simulink library "lib_power_bus2"  (Simulink 10.1)
settings: Solver=VariableStepAuto  StartTime=0.0  StopTime=10.0  RelTol=1e-3
undefined symbols (not defined in the file or in its folder): acc_elec_eff, acc_elec_pwr, cs_hi_soc, cs_lo_soc, ess_on
undefined symbols (not defined in the file): logFlag
libraries: sub_lib_models x2
settings Model: Creator=sateeshk  LastModifiedBy=sateeshk
settings Model: ModifiedComment=|
  | mokeefe -- Thu Apr 18 08:38:09 2002 -- Version 1.10
  | saving the model:
  | o "without the model browser open"
  | o with only top-level screen visible
  | o with "fit to view" enabled
  | o with "status bar" off and "toolbar" off
  | o with "prompt to update model history with each save" on
settings Model: ModifiedHistory=|
  | mokeefe -- Thu Apr 18 08:38:09 2002 -- Version 1.10
  | saving the model:
  | o "without the model browser open"
  | o with only top-level screen visible
  | o with "fit to view" enabled
  | o with "status bar" off and "toolbar" off
  | o with "prompt to update model history with each save" on
  | 
  | mokeefe -- Thu Apr 18 08:38:09 2002 -- Version 1.10
  | saving the model:
  | o "without the model browser open"
  | o with only top-level screen visible
  | o with "fit to view" enabled
  | o with "status bar" off and "toolbar" off
  | o with "prompt to update model history with each save" on

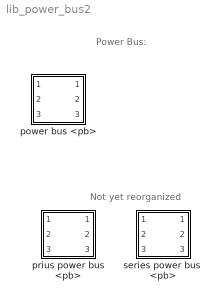
== system lib_power_bus2 ==
  note: Power Bus:
  note: Not yet reorganized
  power bus <pb> : Subsystem  mask(Stand-Alone Power Bus Mask){generalName='pb', logPick=Log, initFileName={}, modCell={}, imgFileName='bdi_pb.jpg', DEBUG=ON}
      mask prompts: generalName "General Name of this Component [char]"; logPick "Log Variables to Workspace?"; initFileName "Initialization File(s) [cell array of char]"; modCell "Modification Cell [2 column cell array of param and val]"; imgFileName "Icon image file name [char--evaluated]"
      mask init:
      | % initialization via m-file script
      | advSACompMaskInit;
      mask TypeOptions logPick: Don't Log | Log
      mask TypeOptions DEBUG: ON | OFF
      mask Display: image(imread(imgFileName))
  prius power bus <pb> : Subsystem
      mask Display: image(imread('bdi_pb.jpg'))
  series power bus  <pb> : Subsystem
      mask Display: image(imread('bdi_pb.jpg'))

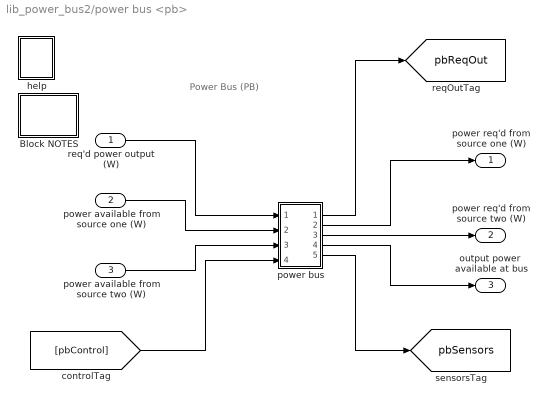
== system lib_power_bus2/power bus <pb> ==
  note: Power Bus (PB)
  req'd power output (W) : Inport
  power available from source one (W) : Inport  Port=2
  power available from source two (W) : Inport  Port=3
  Block NOTES : Subsystem
      mask Display: disp('Block\nNOTES')
  help : Subsystem
      settings: OpenFcn=web(['file:\\\' which('fuel_converter.htm')]);
      mask Display: image(imread('doc_man.jpg'))
  power bus : Subsystem
  power req'd from source one (W) : Outport
  power req'd from source two (W) : Outport  Port=2
  output power  available at bus : Outport  Port=3
  tag scope: pbReqOut=global, pbSensors=global
  wires:
  req'd power output (W)/1 -> power bus/1(power out req)
  power available from source one (W)/1 -> power bus/2(power available from source one)
  power available from source two (W)/1 -> power bus/3(power available from source two)
  [pbControl] -> power bus/4(control)
  power bus/1(required out) -> [pbReqOut]
  power bus/2(power in req from  source one) -> power req'd from source one (W)/1
  power bus/3(power in req from  source two) -> power req'd from source two (W)/1
  power bus/4(power out available) -> output power  available at bus/1
  power bus/5(sensors) -> [pbSensors]

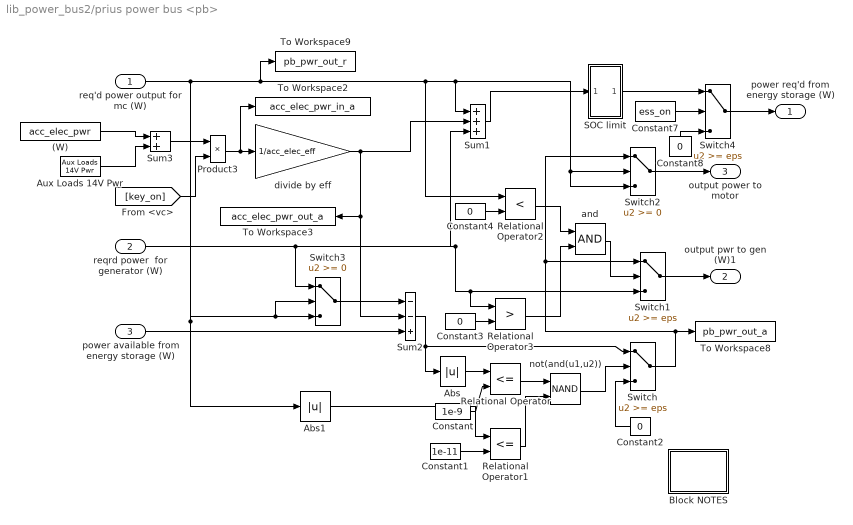
== system lib_power_bus2/prius power bus <pb> ==
  req'd power output for mc (W) : Inport
  reqrd power  for generator (W) : Inport  Port=2
  power available from energy storage (W) : Inport  Port=3
  (W) : Constant  Value=acc_elec_pwr
  Abs : Abs  SaturateOnIntegerOverflow=on
  Abs1 : Abs  SaturateOnIntegerOverflow=on
  Aux Loads 14V Pwr : sub_lib_models/Aux Loads 14V Pwr
      settings: RTWFcnNameOpts=Auto  RTWFileNameOpts=Auto
  Block NOTES : Subsystem
      mask Display: disp('Block\nNOTES')
  Constant : Constant  Value=1e-9
  Constant1 : Constant  Value=1e-11
  Constant{2..4,8} (4 alike) : Constant  Value=0
  Constant7 : Constant  Value=ess_on
  Product3 : Product  SaturateOnIntegerOverflow=on
  Relational Operator : RelationalOperator  Operator=<=  RndMeth=Nearest  InputSameDT=on
  Relational Operator1 : RelationalOperator  Operator=<=  RndMeth=Nearest  InputSameDT=on
  Relational Operator2 : RelationalOperator  Operator=<  RndMeth=Nearest  InputSameDT=on
  Relational Operator3 : RelationalOperator  Operator=>  RndMeth=Nearest  InputSameDT=on
  SOC limit : Subsystem
  Sum1 : Sum  Inputs=+++  SaturateOnIntegerOverflow=on
  Sum2 : Sum  Inputs=--+  SaturateOnIntegerOverflow=on
  Sum3 : Sum  SaturateOnIntegerOverflow=on
  Switch : Switch  Threshold=eps  SaturateOnIntegerOverflow=on  InputSameDT=on
  Switch1 : Switch  Threshold=eps  SaturateOnIntegerOverflow=on  InputSameDT=on
  Switch2 : Switch  SaturateOnIntegerOverflow=on  InputSameDT=on
  Switch3 : Switch  SaturateOnIntegerOverflow=on  InputSameDT=on
  Switch4 : Switch  Threshold=eps  SaturateOnIntegerOverflow=on  InputSameDT=on
  To Workspace2 : ToWorkspace  VariableName=acc_elec_pwr_in_a  SampleTime=-1
  To Workspace3 : ToWorkspace  VariableName=acc_elec_pwr_out_a  SampleTime=-1
  To Workspace8 : ToWorkspace  VariableName=pb_pwr_out_a  SampleTime=-1
  To Workspace9 : ToWorkspace  VariableName=pb_pwr_out_r  SampleTime=-1
  and : Logic
  divide by eff : Gain  Gain=1/acc_elec_eff  SaturateOnIntegerOverflow=on
  not(and(u1,u2)) : Logic  Operator=NAND
  power req'd from energy storage (W) : Outport
  output pwr to gen (W)1 : Outport  Port=2
  output power to motor : Outport  Port=3
  wires:
  and/1 -> Switch1/2
  Relational Operator3/1 -> and/2
  Relational Operator2/1 -> and/1
  Constant4/1 -> Relational Operator2/2
  Constant3/1 -> Relational Operator3/2
  Constant8/1 -> Switch4/3
  Constant7/1 -> Switch4/2
  Switch4/1 -> power req'd from energy storage (W)/1
  SOC limit/1(limited pwr req from ess (W)) -> Switch4/1
  Sum1/1 -> SOC limit/1(pwr req to  ess)
  Switch/1 -> Switch2/1, Switch1/1, To Workspace8/1
  reqrd power  for generator (W)/1 -> Switch3/1, Switch1/3, Relational Operator3/1, Sum1/3
  Switch3/1 -> Sum2/1
  Switch1/1 -> output pwr to gen (W)1/1
  Switch2/1 -> output power to motor/1
  Constant1/1 -> Relational Operator1/2
  Relational Operator1/1 -> not(and(u1,u2))/2
  Abs1/1 -> Relational Operator1/1
  Constant/1 -> Relational Operator/2
  Relational Operator/1 -> not(and(u1,u2))/1
  not(and(u1,u2))/1 -> Switch/2
  Constant2/1 -> Switch/3
  Abs/1 -> Relational Operator/1
  Sum2/1 -> Switch/1, Abs/1
  power available from energy storage (W)/1 -> Sum2/3
  Product3/1 -> To Workspace2/1, divide by eff/1
  divide by eff/1 -> Sum1/2, To Workspace3/1, Sum2/2
  [key_on] -> Product3/2
  req'd power output for mc (W)/1 -> Switch3/2, Switch3/3, Abs1/1, Relational Operator2/1, Switch2/2, Switch2/3, Sum1/1, To Workspace9/1
  Sum3/1 -> Product3/1
  (W)/1 -> Sum3/1
  Aux Loads 14V Pwr/1 -> Sum3/2

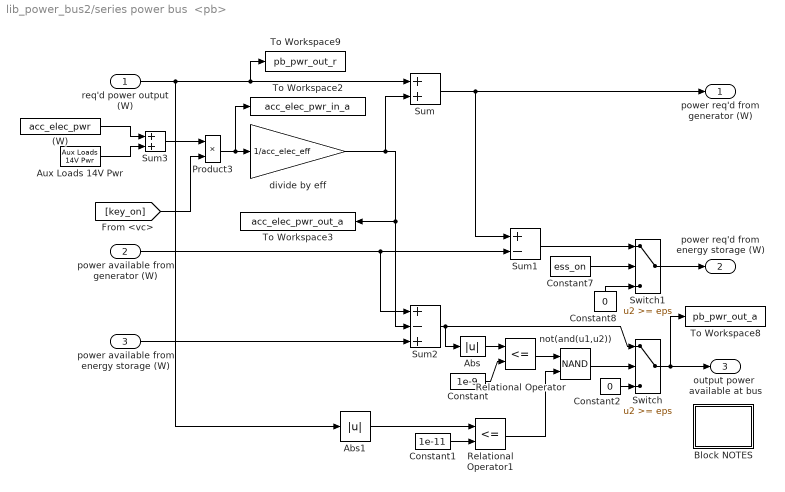
== system lib_power_bus2/series power bus  <pb> ==
  req'd power output (W) : Inport
  power available from generator (W) : Inport  Port=2
  power available from energy storage (W) : Inport  Port=3
  (W) : Constant  Value=acc_elec_pwr
  Abs : Abs  SaturateOnIntegerOverflow=on
  Abs1 : Abs  SaturateOnIntegerOverflow=on
  Aux Loads 14V Pwr : sub_lib_models/Aux Loads 14V Pwr
      settings: RTWFcnNameOpts=Auto  RTWFileNameOpts=Auto
  Block NOTES : Subsystem
      mask Display: disp('Block\nNOTES')
  Constant : Constant  Value=1e-9
  Constant1 : Constant  Value=1e-11
  Constant2 : Constant  Value=0
  Constant7 : Constant  Value=ess_on
  Constant8 : Constant  Value=0
  Product3 : Product  SaturateOnIntegerOverflow=on
  Relational Operator : RelationalOperator  Operator=<=  RndMeth=Nearest  InputSameDT=on
  Relational Operator1 : RelationalOperator  Operator=<=  RndMeth=Nearest  InputSameDT=on
  Sum : Sum  SaturateOnIntegerOverflow=on
  Sum1 : Sum  Inputs=+-  SaturateOnIntegerOverflow=on
  Sum2 : Sum  Inputs=+-+  SaturateOnIntegerOverflow=on
  Sum3 : Sum  SaturateOnIntegerOverflow=on
  Switch : Switch  Threshold=eps  SaturateOnIntegerOverflow=on  InputSameDT=on
  Switch1 : Switch  Threshold=eps  SaturateOnIntegerOverflow=on  InputSameDT=on
  To Workspace2 : ToWorkspace  VariableName=acc_elec_pwr_in_a  SampleTime=-1
  To Workspace3 : ToWorkspace  VariableName=acc_elec_pwr_out_a  SampleTime=-1
  To Workspace8 : ToWorkspace  VariableName=pb_pwr_out_a  SampleTime=-1
  To Workspace9 : ToWorkspace  VariableName=pb_pwr_out_r  SampleTime=-1
  divide by eff : Gain  Gain=1/acc_elec_eff  SaturateOnIntegerOverflow=on
  not(and(u1,u2)) : Logic  Operator=NAND
  power req'd from generator (W) : Outport
  power req'd from energy storage (W) : Outport  Port=2
  output power  available at bus : Outport  Port=3
  wires:
  Constant8/1 -> Switch1/3
  Constant7/1 -> Switch1/2
  Switch1/1 -> power req'd from energy storage (W)/1
  Sum1/1 -> Switch1/1
  Constant/1 -> Relational Operator/2
  Abs/1 -> Relational Operator/1
  Sum2/1 -> Switch/1, Abs/1
  Switch/1 -> output power  available at bus/1, To Workspace8/1
  Constant1/1 -> Relational Operator1/2
  Abs1/1 -> Relational Operator1/1
  Relational Operator1/1 -> not(and(u1,u2))/2
  not(and(u1,u2))/1 -> Switch/2
  Constant2/1 -> Switch/3
  power available from energy storage (W)/1 -> Sum2/3
  Relational Operator/1 -> not(and(u1,u2))/1
  power available from generator (W)/1 -> Sum1/2, Sum2/1
  Product3/1 -> To Workspace2/1, divide by eff/1
  [key_on] -> Product3/2
  Sum/1 -> power req'd from generator (W)/1, Sum1/1
  req'd power output (W)/1 -> To Workspace9/1, Sum/1, Abs1/1
  divide by eff/1 -> Sum/2, Sum2/2, To Workspace3/1
  Sum3/1 -> Product3/1
  (W)/1 -> Sum3/1
  Aux Loads 14V Pwr/1 -> Sum3/2

== system lib_power_bus2/power bus <pb>/Block NOTES ==
  note: This block models the internal combustion engine, and includes inertia effects,
      | performance limits, accessory loads, and temperature transient effects on fuel
      | use, engine-out emissions, and catalyst efficiency.  There are 'leads' to the
      | engine controller here, which controller determines whether the engine is on.

== system lib_power_bus2/power bus <pb>/help ==

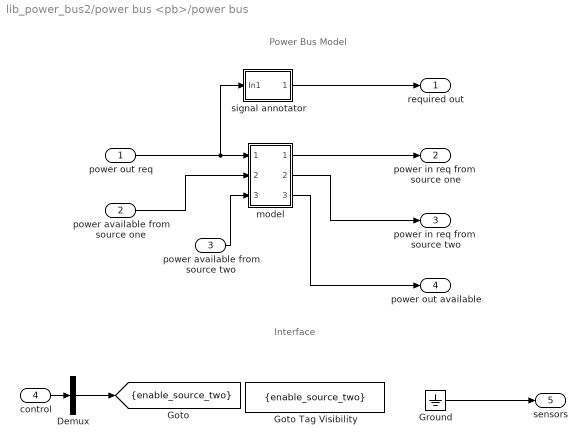
== system lib_power_bus2/power bus <pb>/power bus ==
  note: Interface
  note: Power Bus Model
  power out req : Inport
  power available from source one : Inport  Port=2
  power available from source two : Inport  Port=3
  control : Inport  Port=4
  Demux : Demux  Outputs=1
  Goto Tag Visibility : GotoTagVisibility  GotoTag=enable_source_two
  Ground : Ground
  model : Subsystem
  signal annotator : Subsystem
  required out : Outport
  power in req from  source one : Outport  Port=2
  power in req from  source two : Outport  Port=3
  power out available : Outport  Port=4
  sensors : Outport  Port=5
  tag scope: enable_source_two=scoped
  wires:
  model/1(power req'd from generator (W)) -> power in req from  source one/1
  power out req/1 -> model/1(req'd power output (W)), signal annotator/1(In1)
  model/2(power req'd from energy storage (W)) -> power in req from  source two/1
  power available from source one/1 -> model/2(power available from generator (W))
  model/3(output power  available at bus) -> power out available/1
  power available from source two/1 -> model/3(power available from energy storage (W))
  signal annotator/1(Out1) -> required out/1
  control/1 -> Demux/1
  Demux/1 -> [enable_source_two]
  Ground/1 -> sensors/1

== system lib_power_bus2/prius power bus <pb>/Block NOTES ==
  note: This power bus requires power from (or distributes power to)
      | the generator first, taking the balance from the energy
      | storage system.

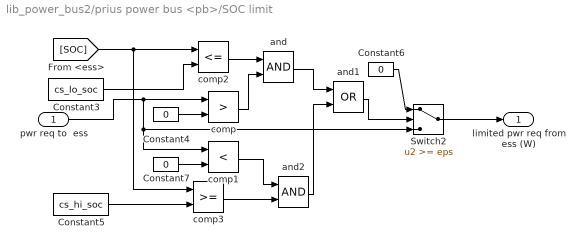
== system lib_power_bus2/prius power bus <pb>/SOC limit ==
  pwr req to  ess : Inport
  Constant3 : Constant  Value=cs_lo_soc
  Constant4 : Constant  Value=0
  Constant5 : Constant  Value=cs_hi_soc
  Constant6 : Constant  Value=0
  Constant7 : Constant  Value=0
  Switch2 : Switch  Threshold=eps  SaturateOnIntegerOverflow=on  InputSameDT=on
  and : Logic
  and1 : Logic  Operator=OR
  and2 : Logic
  comp : RelationalOperator  Operator=>  RndMeth=Nearest  InputSameDT=on
  comp1 : RelationalOperator  Operator=<  RndMeth=Nearest  InputSameDT=on
  comp2 : RelationalOperator  Operator=<=  RndMeth=Nearest  InputSameDT=on
  comp3 : RelationalOperator  RndMeth=Nearest  InputSameDT=on
  limited pwr req from ess (W) : Outport  InitialOutput=0
  wires:
  Switch2/1 -> limited pwr req from ess (W)/1
  comp2/1 -> and/1
  Constant3/1 -> comp2/2
  and/1 -> and1/1
  and1/1 -> Switch2/2
  [SOC] -> comp2/1, comp3/1
  comp/1 -> and/2
  comp1/1 -> and2/1
  pwr req to  ess/1 -> comp/1, comp1/1, Switch2/3
  Constant6/1 -> Switch2/1
  Constant5/1 -> comp3/2
  comp3/1 -> and2/2
  and2/1 -> and1/2
  Constant4/1 -> comp/2
  Constant7/1 -> comp1/2

== system lib_power_bus2/series power bus  <pb>/Block NOTES ==
  note: This power bus requires power from (or distributes power to)
      | the generator first, taking the balance from the energy
      | storage system.

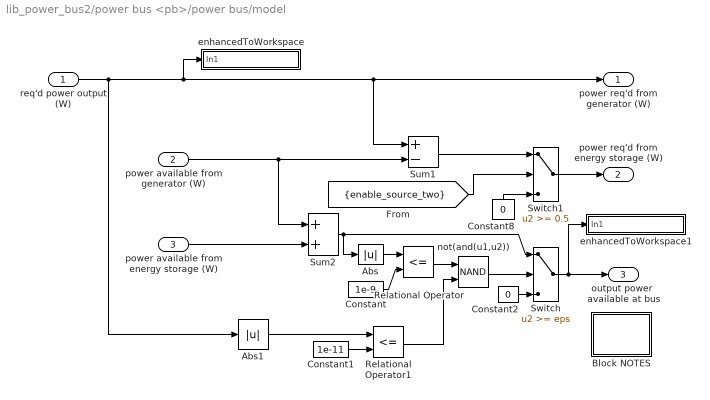
== system lib_power_bus2/power bus <pb>/power bus/model ==
  req'd power output (W) : Inport
  power available from generator (W) : Inport  Port=2
  power available from energy storage (W) : Inport  Port=3
  Abs : Abs  SaturateOnIntegerOverflow=on
  Abs1 : Abs  SaturateOnIntegerOverflow=on
  Block NOTES : Subsystem
      mask Display: disp('Block\nNOTES')
  Constant : Constant  Value=1e-9
  Constant1 : Constant  Value=1e-11
  Constant2 : Constant  Value=0
  Constant8 : Constant  Value=0
  Relational Operator : RelationalOperator  Operator=<=  RndMeth=Nearest  InputSameDT=on
  Relational Operator1 : RelationalOperator  Operator=<=  RndMeth=Nearest  InputSameDT=on
  Sum1 : Sum  Inputs=+-  SaturateOnIntegerOverflow=on
  Sum2 : Sum  SaturateOnIntegerOverflow=on
  Switch : Switch  Threshold=eps  SaturateOnIntegerOverflow=on  InputSameDT=on
  Switch1 : Switch  Threshold=0.5  SaturateOnIntegerOverflow=on  InputSameDT=on
  enhancedToWorkspace : Subsystem  TreatAsAtomicUnit=on  mask(enhancedToWorkspace){generalName=generalName, specificName=pwr_out_r, logFlag=logFlag}
      mask prompts: generalName "General Name [char-evaluated]"; specificName "Specific Name [char-literal]"; logFlag "Enable flag (1=on,0=off)"
      mask help: A wrapper for the Simulink "To Workspace" block that allows you to evaluate the name of the variable to log to workspace. This is useful to avoid the double logging errors that occur when you pull in two library models that attempt to log to the same variable.
      mask init:
      | enhancedToWsMaker
      settings: CopyFcn=breakLinkCopyFcn  ParentCloseFcn=breakLinkParCloseFcn
      mask Help:
      | <h2>Enhanced To Workspace Block</h2>
      | <h3>Parameters</h3>
      | <UL>
      | <li><b>General Name:</b> This is the more general name of the variable. Variables are saved to the workspace as <i>generalName_specificName</i>. Note that this is an evaluated variable. If you would like to type in the value directly, it must be surrounded with single quotes. Otherwise you can input the name of a variable containing a char string.</li>
      | <li><b>Specific Name:</b> This is the specific name of the variable. Note that this is input as a char literal (i.e., you don't need quotes).</li>
      | <li><b>Enable Flag:</b> This flag should have the value of 0 or 1. If 0, the variable will not be logged to the workspace. If 1, the variable will be logged. This is done so that variable logging can be turned off to improve speed.</li>
      | </ul>
      | <h3>Overview</h3>
      | <p>The enhanced to workspace block was put together to allow one to dynamically resolve variable names at run time in simulink. This is most powerful when used in conjunction with a masked subsystem to allow multiple instances of that masked subsytem to be used in the same model. The strategy is to set the generalName in the block mask which will allow the block to change the general name for all variable logging on the fly.
      | <h3>Helper Files</h3>
      | <p>Three m-files are required by the enhancedToWorkspace block. These files are located in the &lt; ADVISOR root &gt;/GUI directory :
      | <ul>
      | <li><i>enhancedToWsMaker.m</i> This file runs the mask initialization for the block</li>
      | <li><i>breakLinkCopyFcn.m</i> This file is used by the block callback when the simulink block is copied. It is necessary to break the link to the enhancedToWorkspace similar to the To Workspace block in order for it to be able to configure itself. (Try copying simulink's To Workspace block--it is impossible to make a link)</li>
      | <li><i>breakLinkParCloseFcn.m</i> This file is similar to the breakLinkCopyFcn and is used when a parent system is closed</li>
      | </ul>
      | <hr>
      | 
      | <p>Created 2003-Jan-21, Michael Patrick O'Keefe, NREL</p>
      | 
      | <!--
      | <VARDEF>
      | <H3>var_name</H3>
      | <UL>
      | <LI><B>data type</B> data type here</LI>
      | <LI><B>units</B> units here</LI>
      | <LI><B>vehicle type</B> vehicle type here</LI>
      | <LI><B>description</B> description here</LI>
      | </UL>
      | </VARDEF>
      | -->
      mask Display: disp([generalName,'_',specificName])
  enhancedToWorkspace1 : Subsystem  TreatAsAtomicUnit=on  mask(enhancedToWorkspace){generalName=generalName, specificName=pwr_out_a, logFlag=logFlag}
      mask prompts: generalName "General Name [char-evaluated]"; specificName "Specific Name [char-literal]"; logFlag "Enable flag (1=on,0=off)"
      mask help: A wrapper for the Simulink "To Workspace" block that allows you to evaluate the name of the variable to log to workspace. This is useful to avoid the double logging errors that occur when you pull in two library models that attempt to log to the same variable.
      mask init:
      | enhancedToWsMaker
      settings: CopyFcn=breakLinkCopyFcn  ParentCloseFcn=breakLinkParCloseFcn
      mask Help:
      | <h2>Enhanced To Workspace Block</h2>
      | <h3>Parameters</h3>
      | <UL>
      | <li><b>General Name:</b> This is the more general name of the variable. Variables are saved to the workspace as <i>generalName_specificName</i>. Note that this is an evaluated variable. If you would like to type in the value directly, it must be surrounded with single quotes. Otherwise you can input the name of a variable containing a char string.</li>
      | <li><b>Specific Name:</b> This is the specific name of the variable. Note that this is input as a char literal (i.e., you don't need quotes).</li>
      | <li><b>Enable Flag:</b> This flag should have the value of 0 or 1. If 0, the variable will not be logged to the workspace. If 1, the variable will be logged. This is done so that variable logging can be turned off to improve speed.</li>
      | </ul>
      | <h3>Overview</h3>
      | <p>The enhanced to workspace block was put together to allow one to dynamically resolve variable names at run time in simulink. This is most powerful when used in conjunction with a masked subsystem to allow multiple instances of that masked subsytem to be used in the same model. The strategy is to set the generalName in the block mask which will allow the block to change the general name for all variable logging on the fly.
      | <h3>Helper Files</h3>
      | <p>Three m-files are required by the enhancedToWorkspace block. These files are located in the &lt; ADVISOR root &gt;/GUI directory :
      | <ul>
      | <li><i>enhancedToWsMaker.m</i> This file runs the mask initialization for the block</li>
      | <li><i>breakLinkCopyFcn.m</i> This file is used by the block callback when the simulink block is copied. It is necessary to break the link to the enhancedToWorkspace similar to the To Workspace block in order for it to be able to configure itself. (Try copying simulink's To Workspace block--it is impossible to make a link)</li>
      | <li><i>breakLinkParCloseFcn.m</i> This file is similar to the breakLinkCopyFcn and is used when a parent system is closed</li>
      | </ul>
      | <hr>
      | 
      | <p>Created 2003-Jan-21, Michael Patrick O'Keefe, NREL</p>
      | 
      | <!--
      | <VARDEF>
      | <H3>var_name</H3>
      | <UL>
      | <LI><B>data type</B> data type here</LI>
      | <LI><B>units</B> units here</LI>
      | <LI><B>vehicle type</B> vehicle type here</LI>
      | <LI><B>description</B> description here</LI>
      | </UL>
      | </VARDEF>
      | -->
      mask Display: disp([generalName,'_',specificName])
  not(and(u1,u2)) : Logic  Operator=NAND
  power req'd from generator (W) : Outport
  power req'd from energy storage (W) : Outport  Port=2
  output power  available at bus : Outport  Port=3
  wires:
  req'd power output (W)/1 -> power req'd from generator (W)/1, Sum1/1, enhancedToWorkspace/1(In1), Abs1/1
  power available from generator (W)/1 -> Sum1/2, Sum2/1
  Relational Operator/1 -> not(and(u1,u2))/1
  Constant2/1 -> Switch/3
  not(and(u1,u2))/1 -> Switch/2
  Relational Operator1/1 -> not(and(u1,u2))/2
  Abs1/1 -> Relational Operator1/1
  Constant1/1 -> Relational Operator1/2
  Switch/1 -> output power  available at bus/1, enhancedToWorkspace1/1(In1)
  Sum2/1 -> Abs/1, Switch/1
  Abs/1 -> Relational Operator/1
  Constant/1 -> Relational Operator/2
  Sum1/1 -> Switch1/1
  Switch1/1 -> power req'd from energy storage (W)/1
  [enable_source_two] -> Switch1/2
  Constant8/1 -> Switch1/3
  power available from energy storage (W)/1 -> Sum2/2

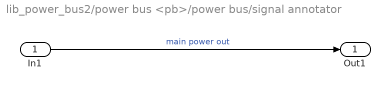
== system lib_power_bus2/power bus <pb>/power bus/signal annotator ==
  In1 : Inport
  Out1 : Outport
  wires:
  In1/1 -> Out1/1  "main power out"

== system lib_power_bus2/power bus <pb>/power bus/model/Block NOTES ==
  note: This power bus requires power from (or distributes power to)
      | the generator first, taking the balance from the energy
      | storage system.

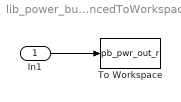
== system lib_power_bus2/power bus <pb>/power bus/model/enhancedToWorkspace ==
  In1 : Inport
  To Workspace : ToWorkspace  VariableName=pb_pwr_out_r  SampleTime=-1
  wires:
  In1/1 -> To Workspace/1

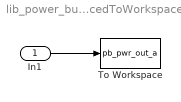
== system lib_power_bus2/power bus <pb>/power bus/model/enhancedToWorkspace1 ==
  In1 : Inport
  To Workspace : ToWorkspace  VariableName=pb_pwr_out_a  SampleTime=-1
  wires:
  In1/1 -> To Workspace/1
